simulink model "DFT_Ex4"  (R2023a)
settings: Solver=VariableStepAuto  StartTime=0.0  StopTime=0.5  RelTol=1e-3
undefined symbols (not defined in the file): None, S, vsva2197, xcvc1902
libraries: aieUtilities x4, dspsrcs4 x2, aieDSP x1, vmcUtilities x1
settings Model: Creator=sdegala  LastModifiedBy=robg
settings ModelReferenceCC: EnableRefExpFcnMdlSchedulingChecks=on

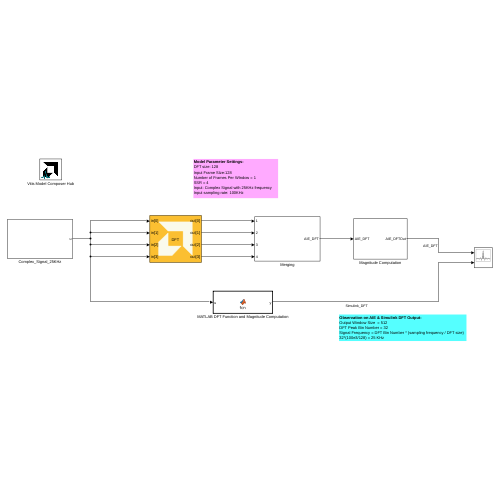
[thumbnail: Simulink's stored preview of the top-level diagram]
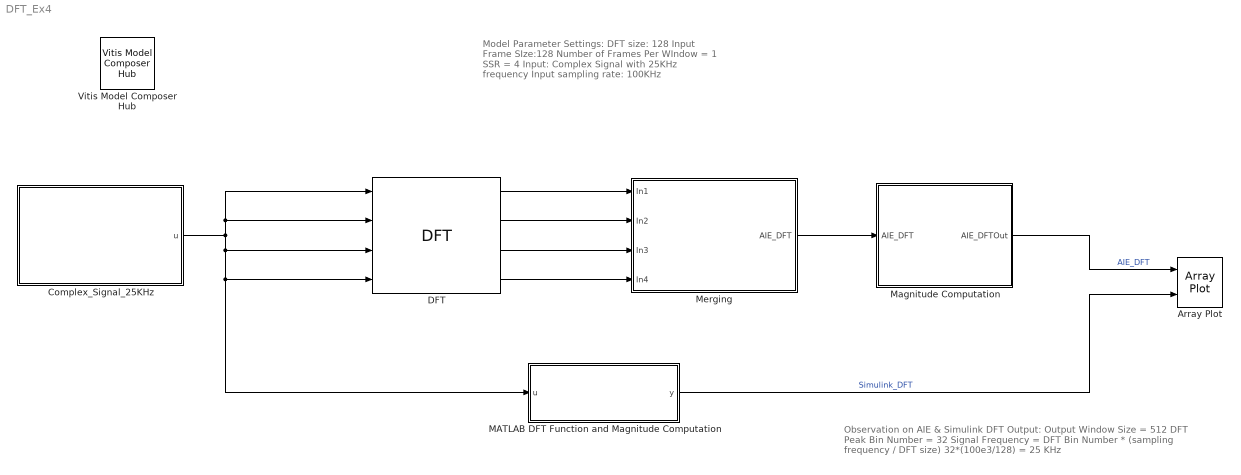
== system DFT_Ex4 ==
  note: Model Parameter Settings:
      | DFT size: 128
      | Input Frame SIze:128
      | Number of Frames Per WIndow = 1
      | SSR = 4
      | Input: Complex Signal with 25KHz frequency
      | Input sampling rate: 100KHz
  note: Observation on AIE & Simulink DFT Output:
      | Output Window Size = 512
      | DFT Peak Bin Number = 32
      | Signal Frequency = DFT Bin Number * (sampling frequency / DFT size)
      | 32*(100e3/128) = 25 KHz
  Array Plot : ArrayPlot  NumInputPorts=2  WindowPosition=[1.000000,1.000000,1280.000000,744.000000,]  Visible=on  ScopeFrameLocation=window  YLimits=[-160 1440]  ShowLegend=on
  Complex_Signal_25KHz : Subsystem
  DFT : aieDSP/DFT  data_type=cint16  twiddle_type=cint16  point_size=128  num_frames=1  shift_val=0  rnd_mode=Floor  ssr=4  sat_mode=0-None  casc_length=1  AIE_VARIANT=1  blockJsonConstraints=[]  blockJsonConstraintsInternal=[]  spec=vmc_dft.json  SerializedMaskParamNames=[]  SerializedMaskParamValues=[]  SerializedMaskParamVisibilities=[]  block_type=DFT  SerializedMaskParamDataypes=typename|typename|uint|uint|uint|uint|uint|uint|uint|uint  SerializedMaskParamEnumStrArr=0|0|0|0|0|Floor,Ceiling,Round to positive infinity,Round to negative infinity,Round symmetrical to infinity,Round symmetrical to zero,Round convergent to even,Round convergent to odd|0|0-None,1-Asymmetric,3-Symmetric|0|0  SerializedMaskParamEnumValArr=0|0|0|0|0|0,1,2,3,4,5,6,7|0|0,1,3|0|0  SerializedMaskParamVectorArr=0|0|0|0|0|0|0|0|0|0
  MATLAB DFT Function and Magnitude Computation : MATLAB Function  TreatAsAtomicUnit=on
  Magnitude Computation : Subsystem
  Merging : Subsystem
  Vitis Model Composer Hub : vmcUtilities/Vitis Model Composer Hub  Tag=genX  CodeGeneration=off  StartColumn=1  NumberOfColumns=1  TargetDirectory=./code  exportDesign=off  analyzeDesign=off  validateDesignOnHw=off  ExportType=AI Engines  IpVendor=xilinx.com  IpLibrary=hls  IpVersion=1.0  IpHWLanguage=Verilog  AieCompilerOptions={}  AieSimulatorOptions={}  CreateTestbench=off  TestbenchStackSize=10  RunRtlSim=off  RunCSim=off  RunAieSim=off  AieSimTimeout=50000  RunAieSimProfiling=off  LaunchVitisAnalyzer=off  PlotOutput=off  RunX86Sim=off  X86SimTimeout=10  GenHwImage=off  GenLibadfXo=off  GenHwValidationCode=off  PlatformType=Not Specified  HwSystemType=Baremetal  HwValidationTarget=hw  ProjDevice=xcvc1902-vsva2197-1LP-e-S  ProjDevicePart=xcvc1902-vsva2197-1LP-e-S  AIEType=AIE  SamplePeriod=-1  ClockFrequency=200  DataPathParallelism=1  xilinxfamily=versalaicore  part=xcvc1902  speed=-1LP-e-S  package=vsva2197  directory=./code  testbench=off  incr_netlist=off  synthesis_tool=Vivado  clock_wrapper=Clock Enables  dbl_ovrd=According to Block Masks  dcm_input_clock_period=10  sysclk_period=10  simulink_period=1  eval_field=0  LogFileName=''  NThreads=4
  wires:
  Magnitude Computation/1(AIE_DFTOut) -> Array Plot/1  "AIE_DFT"
  MATLAB DFT Function and Magnitude Computation/1(y) -> Array Plot/2  "Simulink_DFT"
  DFT/1 -> Merging/1(In1)
  DFT/2 -> Merging/2(In2)
  DFT/3 -> Merging/3(In3)
  DFT/4 -> Merging/4(In4)
  Merging/1(AIE_DFT) -> Magnitude Computation/1(AIE_DFT)
  Complex_Signal_25KHz/1(u) -> DFT/4, MATLAB DFT Function and Magnitude Computation/1(u), DFT/3, DFT/1, DFT/2

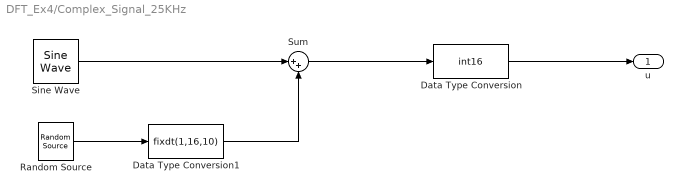
== system DFT_Ex4/Complex_Signal_25KHz ==
  Data Type Conversion : DataTypeConversion  OutDataTypeStr=int16  SaturateOnIntegerOverflow=off  RndMeth=Floor
  Data Type Conversion1 : DataTypeConversion  OutDataTypeStr=fixdt(1,16,10)  SaturateOnIntegerOverflow=off  RndMeth=Floor
  Random Source : dspsrcs4/Random Source  SrcType=Gaussian  NormMethod=Ziggurat  CltLength=12  MinVal=0  MaxVal=1  MeanVal=0  VarVal=0.5  RepMode=Not repeatable  rawSeed=1  IsInherit=off  SampMode=Discrete  SampTime=1/100e3  SampFrame=128  DataType=Single  OutComplex=Real  OutputFrames=off
  Sine Wave : dspsrcs4/Sine Wave  Amplitude=10  Frequency=25e3  Phase=0  SampleMode=Discrete  OutComplex=Complex  CompMethod=Table lookup  TableSize=Speed  SampleTime=1/100e3  SamplesPerFrame=128  ResetState=Restart at time zero  OutputFrames=off  dataType=Fixed-point  wordLen=16  udDataType=sfix(16)  fracBitsMode=User-defined  numFracBits=10  OutDataTypeStr=fixdt(1,16,10)  LastOutDataTypeStr=fixdt(1,16,10)
  Sum : Sum  Inputs=|++
  u : Outport
  wires:
  Sine Wave/1 -> Sum/1
  Data Type Conversion/1 -> u/1
  Random Source/1 -> Data Type Conversion1/1
  Sum/1 -> Data Type Conversion/1
  Data Type Conversion1/1 -> Sum/2

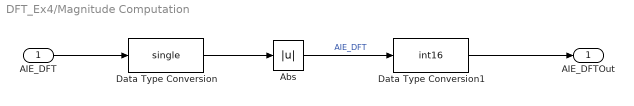
== system DFT_Ex4/Magnitude Computation ==
  AIE_DFT : Inport
  Abs : Abs  SaturateOnIntegerOverflow=off
  Data Type Conversion : DataTypeConversion  OutDataTypeStr=single  SaturateOnIntegerOverflow=off  RndMeth=Floor
  Data Type Conversion1 : DataTypeConversion  OutDataTypeStr=int16  SaturateOnIntegerOverflow=off  RndMeth=Floor
  AIE_DFTOut : Outport
  wires:
  Data Type Conversion/1 -> Abs/1
  Data Type Conversion1/1 -> AIE_DFTOut/1
  Abs/1 -> Data Type Conversion1/1  "AIE_DFT"
  AIE_DFT/1 -> Data Type Conversion/1

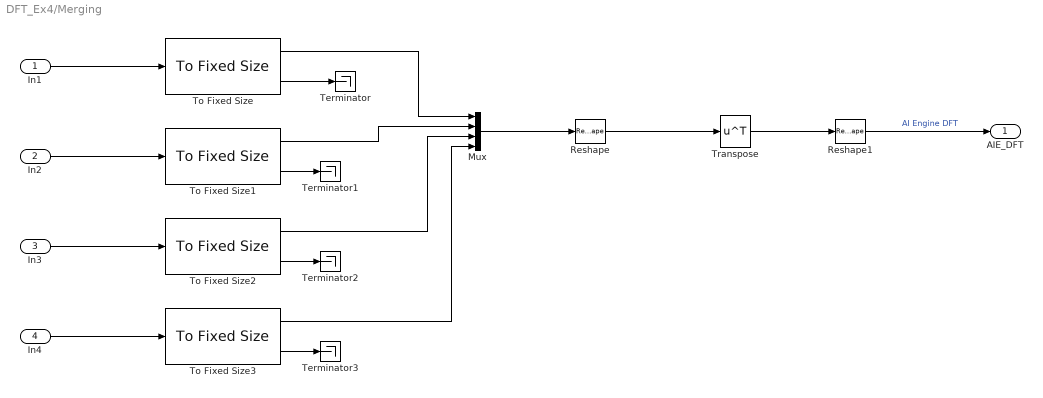
== system DFT_Ex4/Merging ==
  In1 : Inport
  In2 : Inport  Port=2
  In3 : Inport  Port=3
  In4 : Inport  Port=4
  Mux : Mux
  Reshape : Reshape  OutputDimensionality=Customize  OutputDimensions=[32, 4]
  Reshape1 : Reshape  OutputDimensions=[1, 10]
  Terminator{,1..3} (4 alike) : Terminator
  To Fixed Size{,1..3} (4 alike) : aieUtilities/To Fixed Size  Mode=Produce a valid output signal  OutputSize=Inherit: Same as input  CopyMethod=Buffer samples to form output  HasStatusOutput=on
  Transpose : Math  Operator=transpose
  AIE_DFT : Outport
  wires:
  Reshape/1 -> Transpose/1
  To Fixed Size1/2 -> Terminator1/1
  To Fixed Size1/1 -> Mux/2
  In2/1 -> To Fixed Size1/1
  To Fixed Size/2 -> Terminator/1
  Transpose/1 -> Reshape1/1
  To Fixed Size/1 -> Mux/1
  Mux/1 -> Reshape/1
  Reshape1/1 -> AIE_DFT/1  "AI Engine DFT"
  In1/1 -> To Fixed Size/1
  To Fixed Size2/2 -> Terminator2/1
  In4/1 -> To Fixed Size3/1
  To Fixed Size3/1 -> Mux/4
  To Fixed Size3/2 -> Terminator3/1
  In3/1 -> To Fixed Size2/1
  To Fixed Size2/1 -> Mux/3

== matlab function DFT_Ex4/MATLAB DFT Function and Magnitude Computation ==
  data: u input; y output

function y = fcn(u)

DFT_Size = 128; % DFT Size
FramesPerWindow = 1; %No.of Frames Per Window
u = single(u);

X = single(complex(zeros(DFT_Size,FramesPerWindow)));

for m = 1:1:FramesPerWindow
for k = 0:DFT_Size-1
    for n = 0:DFT_Size-1
        X(k+1,m) = X(k+1,m) + u(n+1)*exp(-1i*2*pi*n*k/DFT_Size);
    end
end
end

y = int16(abs(reshape(X,DFT_Size*FramesPerWindow,1)));
